simulink library "SimplusGT"  (R2020a)
settings: Solver=ode45  StartTime=0.0  StopTime=10.0  RelTol=1e-3
undefined symbols (not defined in the file): ang_r, Cf, DiscIntNeverNeededParam, initial, Lc, Lf, m, OtherInputs, P_dc, Sbase, t0, Tm_pu, Ts, V, Vbase, w_droop, w_i, w_pll, w_tau, w_v, Wbase, wc, wfil, x0, Ybase, Zbase
libraries: powerlib x307, $bdroot x1, SimplexPS_2015a x1
(part 5 of 7)

== system SimplusGT/SynchronousMachineFull_SMAVRPSS (dq-Frame System Object) ==
  note: Electrical Circuit
  note: Auxiliary
  note: Matlab System Object
  note: Synchronous machine IN Cyprus 14-bus system with AVR, PSS and GOV.
      |
      | Author(s): Yue Zhu
      |
      | Notes:
      |
      | This model is based on matlab system object.
      |
      | The model is in load convention.
      |
      | The frame transformation between dq and abc is done by simulink blocks, i.e., outside the system object.
  note: The actual current with considering discretization
  Bus Creator : BusCreator  Inputs=7
  Constant2 : Constant  Value=OtherInputs
  Constant5 : Constant  Value=2*pi
  Demux : Demux
  Demux1 : Demux  Outputs=3
  Demux2 : Demux  Outputs=2
  Demux3 : Demux  Outputs=2
  Gain : Gain  Gain=1/Wbase
  Gain1 : Gain  Gain=1/Vbase
  Gain2 : Gain  Gain=Sbase/Vbase
  Gain3 : Gain  Gain=1/(Sbase/Vbase)
  MATLAB System1 : MATLABSystem  System=SimplusGT.Class.SynchronousMachineFull_SMAVRPSS  Ts=Ts  Para=ApparatusPara  ApparatusType=ApparatusType  PowerFlow=PowerFlow  x0=x0  DiscreMethod=DiscreMethod  LinearizationTimes=LinearizationTimes  DirectFeedthrough=DirectFeedthrough  VirtualResistor=DiscreDampingFlag  EquiInitial=true  ElecPortIOs=[ 1, 2 ]  SimulateUsing=Code generation
      mask Type: SimplusGT.Class.SynchronousMachineFull_SMAVRPSS
      mask Display:
      | disp('SynchronousMachineFull_SMAVRPSS');
      | port_label('input',1,'u');
      | port_label('output',1,'y');
  Math Function2 : Math  Operator=mod  SignedPower=on  SaturateOnIntegerOverflow=on
  Mux : Mux  Inputs=2
  Mux1 : Mux  Inputs=3
  Mux2 : Mux
  Mux3 : Mux  Inputs=3
  PQ Calculation (dq-Frame) : Subsystem  AncestorBlock=|
      | SimplusGT/PQ Calculation
      | (dq-Frame)
  R_VD : powerlib/Elements/Three-Phase Series RLC Branch  LConnTagsString=A|B|C  RConnTagsString=A|B|C  BranchType=R  Resistance=DiscreDampingValue*Vbase^2/Sbase  Inductance=1e-3  Capacitance=1e-6  Measurements=None
  "abc -> dq (Power-Invariant)" : Subsystem  AncestorBlock=|
      | SimplusGT/abc -> dq
      | (Power-Invariant)
  "abc -> dq (Power-Invariant)1" : Subsystem  AncestorBlock=|
      | SimplusGT/abc -> dq
      | (Power-Invariant)
  "dq -> abc (Power-Invariant)" : Subsystem  AncestorBlock=|
      | SimplusGT/dq -> abc
      | (Power-Invariant)
  ia : powerlib/Electrical Sources/Controlled Current Source  Initialize=on  Source_Type=AC  Amplitude=0  Phase=0  Frequency=0  Measurements=None
  ia_m : powerlib/Measurements/Current Measurement  PhasorSimulation=off  OutputType=Complex  PSBequivalent=0
  ib : powerlib/Electrical Sources/Controlled Current Source  Initialize=on  Source_Type=AC  Amplitude=0  Phase=0  Frequency=0  Measurements=None
  ib_m : powerlib/Measurements/Current Measurement  PhasorSimulation=off  OutputType=Complex  PSBequivalent=0
  ic : powerlib/Electrical Sources/Controlled Current Source  Initialize=on  Source_Type=AC  Amplitude=0  Phase=0  Frequency=0  Measurements=None
  ic_m : powerlib/Measurements/Current Measurement  PhasorSimulation=off  OutputType=Complex  PSBequivalent=0
  va : powerlib/Measurements/Voltage Measurement  PhasorSimulation=off  OutputType=Complex  PSBequivalent=0
  vb : powerlib/Measurements/Voltage Measurement  PhasorSimulation=off  OutputType=Complex  PSBequivalent=0
  vc : powerlib/Measurements/Voltage Measurement  PhasorSimulation=off  OutputType=Complex  PSBequivalent=0
  a : PMIOPort  Side=Left
  b : PMIOPort  Port=2  Side=Left
  c : PMIOPort  Port=3  Side=Left
  n : PMIOPort  Port=4  Side=Left
  m : Outport
  wires:
  "abc -> dq (Power-Invariant)1"/1(dq) -> [i_dq_t]
  [theta] -> "abc -> dq (Power-Invariant)1"/2(theta)
  [i_abc_t] -> "abc -> dq (Power-Invariant)1"/1(abc)
  Gain3/1 -> [i_abc_t]
  Mux3/1 -> Gain3/1
  ic_m/1 -> Mux3/3
  ib_m/1 -> Mux3/2
  ia_m/1 -> Mux3/1
  Gain2/1 -> Demux1/1
  Gain1/1 -> [v_abc]
  [pq] -> Bus Creator/7  "pq"
  PQ Calculation (dq-Frame)/1(pq) -> [pq]
  [i_dq_t] -> PQ Calculation (dq-Frame)/2(idq)  "i_dq"
  [v_dq] -> PQ Calculation (dq-Frame)/1(vdq)  "v_dq"
  [i_abc] -> Gain2/1
  Demux3/2 -> Mux2/4
  Demux3/1 -> Mux2/3
  Constant2/1 -> Demux3/1
  Mux1/1 -> Gain1/1
  Gain/1 -> Bus Creator/5  "w"
  Bus Creator/1 -> m/1
  [theta] -> Bus Creator/6  "theta"
  [w] -> Gain/1  "w"
  [i_abc_t] -> Bus Creator/4  "i_abc"
  [v_abc] -> Bus Creator/3  "v_abc"
  [i_dq_t] -> Bus Creator/2  "i_dq"
  [v_dq] -> Bus Creator/1  "v_dq"
  Math Function2/1 -> [theta]
  Constant5/1 -> Math Function2/2
  Demux/4 -> Math Function2/1
  Demux1/3 -> ic/1
  vc/1 -> Mux1/3
  MATLAB System1/1 -> Demux/1
  Mux2/1 -> MATLAB System1/1
  "dq -> abc (Power-Invariant)"/1(abc) -> [i_abc]
  [theta] -> "dq -> abc (Power-Invariant)"/2(theta)
  [i_dq] -> "dq -> abc (Power-Invariant)"/1(dq)
  "abc -> dq (Power-Invariant)"/1(dq) -> [v_dq]
  [theta] -> "abc -> dq (Power-Invariant)"/2(theta)
  [v_abc] -> "abc -> dq (Power-Invariant)"/1(abc)
  Demux2/2 -> Mux2/2
  Demux2/1 -> Mux2/1
  [v_dq] -> Demux2/1
  vb/1 -> Mux1/2
  va/1 -> Mux1/1
  Demux1/2 -> ib/1
  Demux1/1 -> ia/1
  Demux/3 -> [w]
  Mux/1 -> [i_dq]
  Demux/1 -> Mux/1
  Demux/2 -> Mux/2
  connections:
  ic_m/LConn1 -- c/RConn1
  ib_m/LConn1 -- b/RConn1
  ia_m/LConn1 -- a/RConn1
  ia_m/RConn1 -- ia/LConn1 -- R_VD/LConn1 -- va/LConn1
  vc/LConn1 -- ic_m/RConn1 -- ic/LConn1 -- R_VD/LConn3
  ib/LConn1 -- ib_m/RConn1 -- vb/LConn1 -- R_VD/LConn2
  ic/RConn1 -- n/RConn1 -- ib/RConn1 -- ia/RConn1 -- R_VD/RConn1 -- R_VD/RConn2 -- R_VD/RConn3 -- vc/LConn2 -- va/LConn2 -- vb/LConn2

== system SimplusGT/SynchronousMachineFull_SMAVRPSSGOV (dq-Frame System Object) ==
  note: Electrical Circuit
  note: Auxiliary
  note: Matlab System Object
  note: Synchronous machine IN Cyprus 14-bus system with AVR, PSS and GOV.
      |
      | Author(s): Yue Zhu
      |
      | Notes:
      |
      | This model is based on matlab system object.
      |
      | The model is in load convention.
      |
      | The frame transformation between dq and abc is done by simulink blocks, i.e., outside the system object.
  note: The actual current with considering discretization
  Bus Creator : BusCreator  Inputs=7
  Constant2 : Constant  Value=OtherInputs
  Constant5 : Constant  Value=2*pi
  Demux : Demux
  Demux1 : Demux  Outputs=3
  Demux2 : Demux  Outputs=2
  Demux3 : Demux  Outputs=2
  Gain : Gain  Gain=1/Wbase
  Gain1 : Gain  Gain=1/Vbase
  Gain2 : Gain  Gain=Sbase/Vbase
  Gain3 : Gain  Gain=1/(Sbase/Vbase)
  MATLAB System : MATLABSystem  System=SimplusGT.Class.SynchronousMachineFull_SMAVRPSSGOV  Ts=Ts  Para=ApparatusPara  ApparatusType=ApparatusType  PowerFlow=PowerFlow  x0=x0  DiscreMethod=DiscreMethod  LinearizationTimes=LinearizationTimes  DirectFeedthrough=DirectFeedthrough  VirtualResistor=DiscreDampingFlag  EquiInitial=true  ElecPortIOs=[ 1, 2 ]  SimulateUsing=Code generation
      mask Type: SimplusGT.Class.SynchronousMachineFull_SMAVRPSSGOV
      mask Display:
      | disp('SynchronousMachineFull_SMAVRPSSGOV');
      | port_label('input',1,'u');
      | port_label('output',1,'y');
  Math Function2 : Math  Operator=mod  SignedPower=on  SaturateOnIntegerOverflow=on
  Mux : Mux  Inputs=2
  Mux1 : Mux  Inputs=3
  Mux2 : Mux
  Mux3 : Mux  Inputs=3
  PQ Calculation (dq-Frame) : Subsystem  AncestorBlock=|
      | SimplusGT/PQ Calculation
      | (dq-Frame)
  R_VD : powerlib/Elements/Three-Phase Series RLC Branch  LConnTagsString=A|B|C  RConnTagsString=A|B|C  BranchType=R  Resistance=DiscreDampingValue*Vbase^2/Sbase  Inductance=1e-3  Capacitance=1e-6  Measurements=None
  "abc -> dq (Power-Invariant)" : Subsystem  AncestorBlock=|
      | SimplusGT/abc -> dq
      | (Power-Invariant)
  "abc -> dq (Power-Invariant)1" : Subsystem  AncestorBlock=|
      | SimplusGT/abc -> dq
      | (Power-Invariant)
  "dq -> abc (Power-Invariant)" : Subsystem  AncestorBlock=|
      | SimplusGT/dq -> abc
      | (Power-Invariant)
  ia : powerlib/Electrical Sources/Controlled Current Source  Initialize=on  Source_Type=AC  Amplitude=0  Phase=0  Frequency=0  Measurements=None
  ia_m : powerlib/Measurements/Current Measurement  PhasorSimulation=off  OutputType=Complex  PSBequivalent=0
  ib : powerlib/Electrical Sources/Controlled Current Source  Initialize=on  Source_Type=AC  Amplitude=0  Phase=0  Frequency=0  Measurements=None
  ib_m : powerlib/Measurements/Current Measurement  PhasorSimulation=off  OutputType=Complex  PSBequivalent=0
  ic : powerlib/Electrical Sources/Controlled Current Source  Initialize=on  Source_Type=AC  Amplitude=0  Phase=0  Frequency=0  Measurements=None
  ic_m : powerlib/Measurements/Current Measurement  PhasorSimulation=off  OutputType=Complex  PSBequivalent=0
  va : powerlib/Measurements/Voltage Measurement  PhasorSimulation=off  OutputType=Complex  PSBequivalent=0
  vb : powerlib/Measurements/Voltage Measurement  PhasorSimulation=off  OutputType=Complex  PSBequivalent=0
  vc : powerlib/Measurements/Voltage Measurement  PhasorSimulation=off  OutputType=Complex  PSBequivalent=0
  a : PMIOPort  Side=Left
  b : PMIOPort  Port=2  Side=Left
  c : PMIOPort  Port=3  Side=Left
  n : PMIOPort  Port=4  Side=Left
  m : Outport
  wires:
  "abc -> dq (Power-Invariant)1"/1(dq) -> [i_dq_t]
  [theta] -> "abc -> dq (Power-Invariant)1"/2(theta)
  [i_abc_t] -> "abc -> dq (Power-Invariant)1"/1(abc)
  Gain3/1 -> [i_abc_t]
  Mux3/1 -> Gain3/1
  ic_m/1 -> Mux3/3
  ib_m/1 -> Mux3/2
  ia_m/1 -> Mux3/1
  Gain2/1 -> Demux1/1
  Gain1/1 -> [v_abc]
  [pq] -> Bus Creator/7  "pq"
  PQ Calculation (dq-Frame)/1(pq) -> [pq]
  [i_dq_t] -> PQ Calculation (dq-Frame)/2(idq)  "i_dq"
  [v_dq] -> PQ Calculation (dq-Frame)/1(vdq)  "v_dq"
  [i_abc] -> Gain2/1
  Demux3/2 -> Mux2/4
  Demux3/1 -> Mux2/3
  Constant2/1 -> Demux3/1
  Mux1/1 -> Gain1/1
  Gain/1 -> Bus Creator/5  "w"
  Bus Creator/1 -> m/1
  [theta] -> Bus Creator/6  "theta"
  [w] -> Gain/1  "w"
  [i_abc_t] -> Bus Creator/4  "i_abc"
  [v_abc] -> Bus Creator/3  "v_abc"
  [i_dq_t] -> Bus Creator/2  "i_dq"
  [v_dq] -> Bus Creator/1  "v_dq"
  Math Function2/1 -> [theta]
  Constant5/1 -> Math Function2/2
  Demux/4 -> Math Function2/1
  Demux1/3 -> ic/1
  vc/1 -> Mux1/3
  MATLAB System/1 -> Demux/1
  Mux2/1 -> MATLAB System/1
  "dq -> abc (Power-Invariant)"/1(abc) -> [i_abc]
  [theta] -> "dq -> abc (Power-Invariant)"/2(theta)
  [i_dq] -> "dq -> abc (Power-Invariant)"/1(dq)
  "abc -> dq (Power-Invariant)"/1(dq) -> [v_dq]
  [theta] -> "abc -> dq (Power-Invariant)"/2(theta)
  [v_abc] -> "abc -> dq (Power-Invariant)"/1(abc)
  Demux2/2 -> Mux2/2
  Demux2/1 -> Mux2/1
  [v_dq] -> Demux2/1
  vb/1 -> Mux1/2
  va/1 -> Mux1/1
  Demux1/2 -> ib/1
  Demux1/1 -> ia/1
  Demux/3 -> [w]
  Mux/1 -> [i_dq]
  Demux/1 -> Mux/1
  Demux/2 -> Mux/2
  connections:
  ic_m/LConn1 -- c/RConn1
  ib_m/LConn1 -- b/RConn1
  ia_m/LConn1 -- a/RConn1
  ia_m/RConn1 -- ia/LConn1 -- R_VD/LConn1 -- va/LConn1
  vc/LConn1 -- ic_m/RConn1 -- ic/LConn1 -- R_VD/LConn3
  ib/LConn1 -- ib_m/RConn1 -- vb/LConn1 -- R_VD/LConn2
  ic/RConn1 -- n/RConn1 -- ib/RConn1 -- ia/RConn1 -- R_VD/RConn1 -- R_VD/RConn2 -- R_VD/RConn3 -- vc/LConn2 -- va/LConn2 -- vb/LConn2

== system SimplusGT/SynchronousMachineFull_SM_GOV (dq-Frame System Object) ==
  note: Electrical Circuit
  note: Auxiliary
  note: Matlab System Object
  note: Synchronous machine IN Cyprus 14-bus system with AVR, PSS and GOV.
      |
      | Author(s): Yue Zhu
      |
      | Notes:
      |
      | This model is based on matlab system object.
      |
      | The model is in load convention.
      |
      | The frame transformation between dq and abc is done by simulink blocks, i.e., outside the system object.
  note: The actual current with considering discretization
  Bus Creator : BusCreator  Inputs=7
  Constant2 : Constant  Value=OtherInputs
  Constant5 : Constant  Value=2*pi
  Demux : Demux
  Demux1 : Demux  Outputs=3
  Demux2 : Demux  Outputs=2
  Demux3 : Demux  Outputs=2
  Gain : Gain  Gain=1/Wbase
  Gain1 : Gain  Gain=1/Vbase
  Gain2 : Gain  Gain=Sbase/Vbase
  Gain3 : Gain  Gain=1/(Sbase/Vbase)
  MATLAB System : MATLABSystem  System=SimplusGT.Class.SynchronousMachineFull_SM_GOV  Ts=Ts  Para=ApparatusPara  ApparatusType=ApparatusType  PowerFlow=PowerFlow  x0=x0  DiscreMethod=DiscreMethod  LinearizationTimes=LinearizationTimes  DirectFeedthrough=DirectFeedthrough  VirtualResistor=DiscreDampingFlag  EquiInitial=true  ElecPortIOs=[ 1, 2 ]  SimulateUsing=Code generation
      mask Type: SimplusGT.Class.SynchronousMachineFull_SM_GOV
      mask Display:
      | disp('SynchronousMachineFull_SM_GOV');
      | port_label('input',1,'u');
      | port_label('output',1,'y');
  Math Function2 : Math  Operator=mod  SignedPower=on  SaturateOnIntegerOverflow=on
  Mux : Mux  Inputs=2
  Mux1 : Mux  Inputs=3
  Mux2 : Mux
  Mux3 : Mux  Inputs=3
  PQ Calculation (dq-Frame) : Subsystem  AncestorBlock=|
      | SimplusGT/PQ Calculation
      | (dq-Frame)
  R_VD : powerlib/Elements/Three-Phase Series RLC Branch  LConnTagsString=A|B|C  RConnTagsString=A|B|C  BranchType=R  Resistance=DiscreDampingValue*Vbase^2/Sbase  Inductance=1e-3  Capacitance=1e-6  Measurements=None
  "abc -> dq (Power-Invariant)" : Subsystem  AncestorBlock=|
      | SimplusGT/abc -> dq
      | (Power-Invariant)
  "abc -> dq (Power-Invariant)1" : Subsystem  AncestorBlock=|
      | SimplusGT/abc -> dq
      | (Power-Invariant)
  "dq -> abc (Power-Invariant)" : Subsystem  AncestorBlock=|
      | SimplusGT/dq -> abc
      | (Power-Invariant)
  ia : powerlib/Electrical Sources/Controlled Current Source  Initialize=on  Source_Type=AC  Amplitude=0  Phase=0  Frequency=0  Measurements=None
  ia_m : powerlib/Measurements/Current Measurement  PhasorSimulation=off  OutputType=Complex  PSBequivalent=0
  ib : powerlib/Electrical Sources/Controlled Current Source  Initialize=on  Source_Type=AC  Amplitude=0  Phase=0  Frequency=0  Measurements=None
  ib_m : powerlib/Measurements/Current Measurement  PhasorSimulation=off  OutputType=Complex  PSBequivalent=0
  ic : powerlib/Electrical Sources/Controlled Current Source  Initialize=on  Source_Type=AC  Amplitude=0  Phase=0  Frequency=0  Measurements=None
  ic_m : powerlib/Measurements/Current Measurement  PhasorSimulation=off  OutputType=Complex  PSBequivalent=0
  va : powerlib/Measurements/Voltage Measurement  PhasorSimulation=off  OutputType=Complex  PSBequivalent=0
  vb : powerlib/Measurements/Voltage Measurement  PhasorSimulation=off  OutputType=Complex  PSBequivalent=0
  vc : powerlib/Measurements/Voltage Measurement  PhasorSimulation=off  OutputType=Complex  PSBequivalent=0
  a : PMIOPort  Side=Left
  b : PMIOPort  Port=2  Side=Left
  c : PMIOPort  Port=3  Side=Left
  n : PMIOPort  Port=4  Side=Left
  m : Outport
  wires:
  "abc -> dq (Power-Invariant)1"/1(dq) -> [i_dq_t]
  [theta] -> "abc -> dq (Power-Invariant)1"/2(theta)
  [i_abc_t] -> "abc -> dq (Power-Invariant)1"/1(abc)
  Gain3/1 -> [i_abc_t]
  Mux3/1 -> Gain3/1
  ic_m/1 -> Mux3/3
  ib_m/1 -> Mux3/2
  ia_m/1 -> Mux3/1
  Gain2/1 -> Demux1/1
  Gain1/1 -> [v_abc]
  [pq] -> Bus Creator/7  "pq"
  PQ Calculation (dq-Frame)/1(pq) -> [pq]
  [i_dq_t] -> PQ Calculation (dq-Frame)/2(idq)  "i_dq"
  [v_dq] -> PQ Calculation (dq-Frame)/1(vdq)  "v_dq"
  [i_abc] -> Gain2/1
  Demux3/2 -> Mux2/4
  Demux3/1 -> Mux2/3
  Constant2/1 -> Demux3/1
  Mux1/1 -> Gain1/1
  Gain/1 -> Bus Creator/5  "w"
  Bus Creator/1 -> m/1
  [theta] -> Bus Creator/6  "theta"
  [w] -> Gain/1  "w"
  [i_abc_t] -> Bus Creator/4  "i_abc"
  [v_abc] -> Bus Creator/3  "v_abc"
  [i_dq_t] -> Bus Creator/2  "i_dq"
  [v_dq] -> Bus Creator/1  "v_dq"
  Math Function2/1 -> [theta]
  Constant5/1 -> Math Function2/2
  Demux/4 -> Math Function2/1
  Demux1/3 -> ic/1
  vc/1 -> Mux1/3
  MATLAB System/1 -> Demux/1
  Mux2/1 -> MATLAB System/1
  "dq -> abc (Power-Invariant)"/1(abc) -> [i_abc]
  [theta] -> "dq -> abc (Power-Invariant)"/2(theta)
  [i_dq] -> "dq -> abc (Power-Invariant)"/1(dq)
  "abc -> dq (Power-Invariant)"/1(dq) -> [v_dq]
  [theta] -> "abc -> dq (Power-Invariant)"/2(theta)
  [v_abc] -> "abc -> dq (Power-Invariant)"/1(abc)
  Demux2/2 -> Mux2/2
  Demux2/1 -> Mux2/1
  [v_dq] -> Demux2/1
  vb/1 -> Mux1/2
  va/1 -> Mux1/1
  Demux1/2 -> ib/1
  Demux1/1 -> ia/1
  Demux/3 -> [w]
  Mux/1 -> [i_dq]
  Demux/1 -> Mux/1
  Demux/2 -> Mux/2
  connections:
  ic_m/LConn1 -- c/RConn1
  ib_m/LConn1 -- b/RConn1
  ia_m/LConn1 -- a/RConn1
  ia_m/RConn1 -- ia/LConn1 -- R_VD/LConn1 -- va/LConn1
  vc/LConn1 -- ic_m/RConn1 -- ic/LConn1 -- R_VD/LConn3
  ib/LConn1 -- ib_m/RConn1 -- vb/LConn1 -- R_VD/LConn2
  ic/RConn1 -- n/RConn1 -- ib/RConn1 -- ia/RConn1 -- R_VD/RConn1 -- R_VD/RConn2 -- R_VD/RConn3 -- vc/LConn2 -- va/LConn2 -- vb/LConn2

== system SimplusGT/Three-Phase Bus ==
  note: Electrical Circuit
  note: Model for a three-phase bus.
      |
      | Author(s): Yitong Li
      |
      | Notes:
      |
      | It is simply a short-cuirt with current measurement. It is used in the toolbox model for highlighting the position of a bus and making the layout clearer.
  Mux : Mux  Inputs=3
  ia : powerlib/Measurements/Current Measurement  PhasorSimulation=off  OutputType=Complex  PSBequivalent=0
  ib : powerlib/Measurements/Current Measurement  PhasorSimulation=off  OutputType=Complex  PSBequivalent=0
  ic : powerlib/Measurements/Current Measurement  PhasorSimulation=off  OutputType=Complex  PSBequivalent=0
  a+ : PMIOPort  Side=Left
  -a : PMIOPort  Port=2  Side=Right
  b+ : PMIOPort  Port=3  Side=Left
  -b : PMIOPort  Port=4  Side=Right
  c+ : PMIOPort  Port=5  Side=Left
  -c : PMIOPort  Port=6  Side=Right
  wires:
  Mux/1 -> [iabc]
  ia/1 -> Mux/1
  ib/1 -> Mux/2
  ic/1 -> Mux/3
  connections:
  ic/RConn1 -- -c/RConn1
  ib/LConn1 -- b+/RConn1
  ib/RConn1 -- -b/RConn1
  ic/LConn1 -- c+/RConn1
  ia/LConn1 -- a+/RConn1
  ia/RConn1 -- -a/RConn1

== system SimplusGT/Three-Phase Signal ==
  note: Three-phase signal generator
      |
      | Author(s): Yitong Li
  Constant : Constant  Value=[ud uq]
  Constant1 : Constant  Value=w
  Constant2 : Constant  Value=theta0
  Constant3 : Constant  Value=2*pi
  Discrete-Time Integrator : DiscreteIntegrator  InitialConditionSource=external  SampleTime=Ts  ICPrevOutput=DiscIntNeverNeededParam  ICPrevScaledInput=DiscIntNeverNeededParam
  Math Function1 : Math  Operator=mod  SignedPower=on  SaturateOnIntegerOverflow=on
  "dq -> abc (Power-Invariant)" : Subsystem
  abc : Outport
  dq : Outport  Port=2
  theta : Outport  Port=3
  wires:
  Discrete-Time Integrator/1 -> Math Function1/1
  "dq -> abc (Power-Invariant)"/1(abc) -> abc/1
  Constant/1 -> "dq -> abc (Power-Invariant)"/1(dq), dq/1
  Math Function1/1 -> "dq -> abc (Power-Invariant)"/2(theta), theta/1
  Constant3/1 -> Math Function1/2
  Constant2/1 -> Discrete-Time Integrator/2
  Constant1/1 -> Discrete-Time Integrator/1

== system SimplusGT/Three-Phase Signal (Advanced) ==
  note: Three-phase signal generator
      |
      | Author(s): Yitong Li
      |
      | Notes:
      |
      | This block has advanced settings.
  Constant : Constant  Value=[ud uq]
  Constant1 : Constant  Value=w
  Constant2 : Constant  Value=theta0
  Constant3 : Constant  Value=2*pi
  Constant4 : Constant  Value=enable_freq_step
  Discrete-Time Integrator : DiscreteIntegrator  InitialConditionSource=external  SampleTime=Ts  ICPrevOutput=DiscIntNeverNeededParam  ICPrevScaledInput=DiscIntNeverNeededParam
  Math Function1 : Math  Operator=mod  SignedPower=on  SaturateOnIntegerOverflow=on
  Product : Product
  Step : Step  Time=time_freq_step  Before=1  After=ratio_freq_step  SampleTime=0
  Switch : Switch  Criteria=u2 > Threshold  Threshold=0.5
  "dq -> abc (Power-Invariant)1" : SimplexPS_2015a/Three-Phase Signal/dq -> abc (Power-Invariant)  SystemSampleTime=-1  Latency=0  AutoFrameSizeCalculation=off
  abc : Outport
  dq : Outport  Port=2
  theta : Outport  Port=3
  wires:
  Constant3/1 -> Math Function1/2
  Constant4/1 -> Switch/2
  Switch/1 -> Discrete-Time Integrator/1
  Constant1/1 -> Product/2, Switch/3
  Constant2/1 -> Discrete-Time Integrator/2
  Product/1 -> Switch/1
  Math Function1/1 -> theta/1, "dq -> abc (Power-Invariant)1"/2
  Constant/1 -> dq/1, "dq -> abc (Power-Invariant)1"/1
  Discrete-Time Integrator/1 -> Math Function1/1
  "dq -> abc (Power-Invariant)1"/1 -> abc/1
  Step/1 -> Product/1

== system SimplusGT/Timer ==
  note: Timer
      |
      | Author(s): Yitong Li
  Constant : Constant
  Discrete-Time Integrator : DiscreteIntegrator  SampleTime=Ts  ICPrevOutput=DiscIntNeverNeededParam  ICPrevScaledInput=DiscIntNeverNeededParam
  Gain : Gain
  Gain1 : Gain  Gain=1/60
  Gain2 : Gain  Gain=1/60
  sec : Outport
  min : Outport  Port=2
  h : Outport  Port=3
  wires:
  Constant/1 -> Discrete-Time Integrator/1
  Discrete-Time Integrator/1 -> Gain/1
  Gain/1 -> Gain1/1, sec/1
  Gain1/1 -> Gain2/1, min/1
  Gain2/1 -> h/1

== system SimplusGT/Two-Phase Bus ==
  note: Electrical Circuit
  note: Model for a two-phase bus.
      |
      | Author(s): Yitong Li
      |
      | Notes:
      |
      | It is simply a short-cuirt with current measurement. It is used in the toolbox model for highlighting the position of a bus and making the layout clearer.
  Mux : Mux  Inputs=2
  ia : powerlib/Measurements/Current Measurement  PhasorSimulation=off  OutputType=Complex  PSBequivalent=0
  ib : powerlib/Measurements/Current Measurement  PhasorSimulation=off  OutputType=Complex  PSBequivalent=0
  a+ : PMIOPort  Side=Left
  -a : PMIOPort  Port=2  Side=Right
  b+ : PMIOPort  Port=3  Side=Left
  -b : PMIOPort  Port=4  Side=Right
  wires:
  Mux/1 -> [iab]
  ia/1 -> Mux/1
  ib/1 -> Mux/2
  connections:
  ib/LConn1 -- b+/RConn1
  ib/RConn1 -- -b/RConn1
  ia/LConn1 -- a+/RConn1
  ia/RConn1 -- -a/RConn1

== system SimplusGT/Voltage Measurement (2ph -> 3ph) ==
  note: Three-phase voltage measurement.
      |
      | Author(s): Yitong Li
      |
      | Notes:
      |
      | vc is calculated from va and vb with assuming that va + vb + vc = 0.
  Add : Sum  Inputs=--+
  Constant : Constant  Value=0
  Mux : Mux  Inputs=3
  va : powerlib/Measurements/Voltage Measurement  PhasorSimulation=off  OutputType=Complex  PSBequivalent=0
  vb : powerlib/Measurements/Voltage Measurement  PhasorSimulation=off  OutputType=Complex  PSBequivalent=0
  a : PMIOPort  Side=Left
  b : PMIOPort  Port=2  Side=Left
  n : PMIOPort  Port=3  Side=Left
  vabc : Outport
  wires:
  Mux/1 -> vabc/1
  va/1 -> Mux/1, Add/1
  vb/1 -> Mux/2, Add/2
  Constant/1 -> Add/3
  Add/1 -> Mux/3
  connections:
  vb/LConn2 -- va/LConn2 -- n/RConn1
  vb/LConn1 -- b/RConn1
  va/LConn1 -- a/RConn1

== system SimplusGT/Voltage Measurement (3ph -> 3ph) ==
  note: Three-phase voltage measurement.
      |
      | Author(s): Yitong Li
  Mux : Mux  Inputs=3
  va : powerlib/Measurements/Voltage Measurement  PhasorSimulation=off  OutputType=Complex  PSBequivalent=0
  vb : powerlib/Measurements/Voltage Measurement  PhasorSimulation=off  OutputType=Complex  PSBequivalent=0
  vc : powerlib/Measurements/Voltage Measurement  PhasorSimulation=off  OutputType=Complex  PSBequivalent=0
  a : PMIOPort  Side=Left
  b : PMIOPort  Port=2  Side=Left
  c : PMIOPort  Port=3  Side=Left
  n : PMIOPort  Port=4  Side=Left
  vabc : Outport
  wires:
  vc/1 -> Mux/3
  Mux/1 -> vabc/1
  va/1 -> Mux/1
  vb/1 -> Mux/2
  connections:
  vb/LConn2 -- va/LConn2 -- vc/LConn2 -- n/RConn1
  vc/LConn1 -- c/RConn1
  vb/LConn1 -- b/RConn1
  va/LConn1 -- a/RConn1

== system SimplusGT/Voltage Disturbance ==
  note: Model for a voltage disturbance.
      |
      | Author(s): Yitong Li
  vabc : Inport
  Controlled Voltage Source : powerlib/Electrical Sources/Controlled Voltage Source  Initialize=on  Source_Type=AC  Amplitude=0  Phase=0  Frequency=0  Measurements=None
  Controlled Voltage Source1 : powerlib/Electrical Sources/Controlled Voltage Source  Initialize=on  Source_Type=AC  Amplitude=0  Phase=0  Frequency=0  Measurements=None
  Controlled Voltage Source2 : powerlib/Electrical Sources/Controlled Voltage Source  Initialize=on  Source_Type=AC  Amplitude=0  Phase=0  Frequency=0  Measurements=None
  Demux : Demux  Outputs=3
  Gain : Gain  Gain=Vbase
  a+ : PMIOPort  Side=Right
  a- : PMIOPort  Port=2  Side=Left
  b+ : PMIOPort  Port=3  Side=Right
  b- : PMIOPort  Port=4  Side=Left
  c+ : PMIOPort  Port=5  Side=Right
  c- : PMIOPort  Port=6  Side=Left
  wires:
  vabc/1 -> Gain/1
  Demux/1 -> Controlled Voltage Source/1
  Demux/2 -> Controlled Voltage Source1/1
  Demux/3 -> Controlled Voltage Source2/1
  Gain/1 -> Demux/1
  connections:
  Controlled Voltage Source2/LConn1 -- c-/RConn1
  Controlled Voltage Source1/RConn1 -- b+/RConn1
  Controlled Voltage Source2/RConn1 -- c+/RConn1
  Controlled Voltage Source/RConn1 -- a+/RConn1
  Controlled Voltage Source/LConn1 -- a-/RConn1
  Controlled Voltage Source1/LConn1 -- b-/RConn1

== system SimplusGT/abc -> alpha//beta (Power-Invariant) ==
  note: Frame transformation from abc to alpha/beta.
      |
      | Author(s): Yitong Li
      |
      | Notes:
      |
      | The transformation is power-invariant.
  abc : Inport
  ->alpha : Fcn  Expr=u(1) - 1/2*u(2) - 1/2*u(3)
  ->beta : Fcn  Expr=0 + sqrt(3)/2*u(2) - sqrt(3)/2*u(3)
  Gain : Gain  Gain=sqrt(2/3)
  Mux2 : Mux  Inputs=2
  albe : Outport
  wires:
  abc/1 -> Gain/1
  Mux2/1 -> albe/1
  Gain/1 -> ->alpha/1, ->beta/1
  ->alpha/1 -> Mux2/1
  ->beta/1 -> Mux2/2

== system SimplusGT/abc -> alpha//beta//0 (Power-Invariant) ==
  note: Frame transformation from abc to alpha/beta/0.
      |
      | Author(s): Yitong Li
      |
      | Notes:
      |
      | The transformation is power-invariant.
  abc : Inport
  ->0 : Fcn  Expr=1/sqrt(2)*u(1) + 1/sqrt(2)*u(2) + 1/sqrt(2)*u(3)
  ->alpha : Fcn  Expr=u(1) - 1/2*u(2) - 1/2*u(3)
  ->beta : Fcn  Expr=0 + sqrt(3)/2*u(2) - sqrt(3)/2*u(3)
  Gain : Gain  Gain=sqrt(2/3)
  Mux2 : Mux  Inputs=3
  albe0 : Outport
  wires:
  ->beta/1 -> Mux2/2
  ->alpha/1 -> Mux2/1
  Gain/1 -> ->alpha/1, ->0/1, ->beta/1
  Mux2/1 -> albe0/1
  abc/1 -> Gain/1
  ->0/1 -> Mux2/3

== system SimplusGT/abc -> dq (Power-Invariant) ==
  note: Frame transformation from abc to dq.
      |
      | Author(s): Yitong Li
      |
      | Notes:
      |
      | The transformation is power-invariant.
      |
      | theta is the angle that d axis leads a axis.
      |
      | q axis leads d axis by 90 degrees.
  abc : Inport
  theta : Inport  Port=2
  ->d : Fcn  Expr=cos(u(4))*u(1) + cos(u(4)-2/3*pi)*u(2) + cos(u(4)-4/3*pi)*u(3)
  ->q : Fcn  Expr=-sin(u(4))*u(1) - sin(u(4)-2/3*pi)*u(2) - sin(u(4)-4/3*pi)*u(3)
  Gain : Gain  Gain=sqrt(2/3)
  Mux5 : Mux  Inputs=2
  Mux6 : Mux  Inputs=2
  dq : Outport
  wires:
  Mux5/1 -> ->q/1, ->d/1
  Mux6/1 -> dq/1
  ->q/1 -> Mux6/2
  theta/1 -> Mux5/2
  Gain/1 -> Mux5/1
  ->d/1 -> Mux6/1
  abc/1 -> Gain/1

== system SimplusGT/abc -> dq (Power-Invariant) (Complex Theta) ==
  abc : Inport
  theta+ : Inport  Port=2
  ->d : Fcn  Expr=cos(u(4))*u(1) + cos(u(4)-2/3*pi)*u(2) + cos(u(4)-4/3*pi)*u(3)
  ->q : Fcn  Expr=-sin(u(4))*u(1) - sin(u(4)-2/3*pi)*u(2) - sin(u(4)-4/3*pi)*u(3)
  Complex to Real-Imag : ComplexToRealImag
  Gain : Gain  Gain=sqrt(2/3)
  Math Function : Math  SignedPower=on  SaturateOnIntegerOverflow=on
  Mux5 : Mux  Inputs=2
  Mux6 : Mux  Inputs=2
  Product : Product
  dq : Outport
  wires:
  ->q/1 -> Mux6/2
  abc/1 -> Gain/1
  Mux5/1 -> ->q/1, ->d/1
  Mux6/1 -> dq/1
  ->d/1 -> Mux6/1
  theta+/1 -> Complex to Real-Imag/1
  Complex to Real-Imag/1 -> Mux5/2
  Complex to Real-Imag/2 -> Math Function/1
  Gain/1 -> Product/1
  Product/1 -> Mux5/1
  Math Function/1 -> Product/2

== system SimplusGT/abc -> dq0 (Power-Invariant) ==
  note: Frame transformation from abc to dq0.
      |
      | Author(s): Yitong Li
      |
      | Notes:
      |
      | The transformation is power-invariant.
      |
      | theta is the angle that dq axis leads abc axis, specifically, d axis leads a axis.
      |
      | q axis leads d axis by 90 degrees. b leads a axis 90 degrees. c leads b 90 degrees.
  abc : Inport
  theta : Inport  Port=2
  ->0 : Fcn  Expr=sqrt(2)/2*u(1) + sqrt(2)/2*u(2) + sqrt(2)/2*u(3)
  ->d : Fcn  Expr=cos(u(4))*u(1) + cos(u(4)-2/3*pi)*u(2) + cos(u(4)-4/3*pi)*u(3)
  ->q : Fcn  Expr=-sin(u(4))*u(1) - sin(u(4)-2/3*pi)*u(2) - sin(u(4)-4/3*pi)*u(3)
  Gain : Gain  Gain=sqrt(2/3)
  Mux1 : Mux  Inputs=2
  Mux2 : Mux  Inputs=3
  dq0 : Outport
  wires:
  ->d/1 -> Mux2/1
  ->q/1 -> Mux2/2
  Gain/1 -> Mux1/1
  abc/1 -> Gain/1
  theta/1 -> Mux1/2
  Mux1/1 -> ->0/1, ->d/1, ->q/1
  Mux2/1 -> dq0/1
  ->0/1 -> Mux2/3

== system SimplusGT/abc->dq (Power-Invariant) (theta_dq) ==
  abc : Inport
  theta_dq : Inport  Port=2
  ->d : Fcn  Expr=cos(u(4))*u(1) + cos(u(4)-2/3*pi)*u(2) + cos(u(4)-4/3*pi)*u(3)
  ->q : Fcn  Expr=-sin(u(4))*u(1) - sin(u(4)-2/3*pi)*u(2) - sin(u(4)-4/3*pi)*u(3)
  Demux : Demux  Outputs=2
  Gain : Gain  Gain=sqrt(2/3)
  Math Function : Math  SignedPower=on  SaturateOnIntegerOverflow=on
  Mux5 : Mux  Inputs=2
  Mux6 : Mux  Inputs=2
  Product : Product
  dq : Outport
  wires:
  Gain/1 -> Product/1
  Math Function/1 -> Product/2
  Mux6/1 -> dq/1
  Mux5/1 -> ->q/1, ->d/1
  ->d/1 -> Mux6/1
  Product/1 -> Mux5/1
  abc/1 -> Gain/1
  ->q/1 -> Mux6/2
  theta_dq/1 -> Demux/1
  Demux/1 -> Mux5/2
  Demux/2 -> Math Function/1

== system SimplusGT/alpha//beta -> abc (Power-Invariant) ==
  note: Frame transformation from alpha/beta to abc.
      |
      | Author(s): Yitong Li
      |
      | Notes:
      |
      | The transformation is power-invariant.
  albe : Inport
  ->a : Fcn  Expr=u(1) + 0
  ->b : Fcn  Expr=-1/2*u(1) + sqrt(3)/2*u(2)
  ->c : Fcn  Expr=-1/2*u(1) - sqrt(3)/2*u(2)
  Gain : Gain  Gain=sqrt(2/3)
  Mux2 : Mux  Inputs=3
  abc : Outport
  wires:
  Gain/1 -> ->a/1, ->c/1, ->b/1
  Mux2/1 -> abc/1
  ->c/1 -> Mux2/3
  ->b/1 -> Mux2/2
  ->a/1 -> Mux2/1
  albe/1 -> Gain/1

== system SimplusGT/alpha//beta -> dq ==
  note: Frame transformation from alpha/beta to dq.
      |
      | Author(s): Yitong Li
      |
      | Notes:
      |
      | theta is the angle that dq axis leads alpha/beta axis, specifically, d axis leads alpha axis.
  albe : Inport
  theta : Inport  Port=2
  ->d : Fcn  Expr=cos(u(3))*u(1) + sin(u(3))*u(2)
  ->q : Fcn  Expr=-sin(u(3))*u(1) + cos(u(3))*u(2)
  Mux5 : Mux  Inputs=2
  Mux6 : Mux  Inputs=2
  dq : Outport
  wires:
  Mux5/1 -> ->q/1, ->d/1
  albe/1 -> Mux5/1
  theta/1 -> Mux5/2
  Mux6/1 -> dq/1
  ->q/1 -> Mux6/2
  ->d/1 -> Mux6/1

== system SimplusGT/alpha//beta//0 -> abc (Power-Invariant) ==
  note: Frame transformation from alpha/beta0 to abc.
      |
      | Author(s): Yitong Li
      |
      | Notes:
      |
      | The transformation is power-invariant.
  albe0 : Inport
  ->a : Fcn  Expr=u(1) + 0 + 1/sqrt(2)*u(3)
  ->b : Fcn  Expr=-1/2*u(1) + sqrt(3)/2*u(2) + 1/sqrt(2)*u(3)
  ->c : Fcn  Expr=-1/2*u(1) - sqrt(3)/2*u(2) + 1/sqrt(2)*u(3)
  Gain : Gain  Gain=sqrt(2/3)
  Mux2 : Mux  Inputs=3
  abc : Outport
  wires:
  Gain/1 -> ->a/1, ->c/1, ->b/1
  ->c/1 -> Mux2/3
  albe0/1 -> Gain/1
  ->a/1 -> Mux2/1
  ->b/1 -> Mux2/2
  Mux2/1 -> abc/1

== system SimplusGT/dq -> abc (Power-Invariant) ==
  note: Frame transformation from dq to abc.
      |
      | Author(s): Yitong Li
      |
      | Notes:
      |
      | The transformation is power-invariant.
      |
      | theta is the angle that dq axis leads alpha/beta axis, specifically, d axis leads alpha axis.
  dq : Inport
  theta : Inport  Port=2
  ->a : Fcn  Expr=cos(u(3))*u(1) - sin(u(3))*u(2)
  ->b : Fcn  Expr=cos(u(3)-2/3*pi)*u(1) - sin(u(3)-2/3*pi)*u(2)
  ->c : Fcn  Expr=cos(u(3)-4/3*pi)*u(1) - sin(u(3)-4/3*pi)*u(2)
  Gain : Gain  Gain=sqrt(2/3)
  Mux5 : Mux  Inputs=2
  Mux6 : Mux  Inputs=3
  abc : Outport
  wires:
  theta/1 -> Mux5/2
  Mux5/1 -> ->c/1, ->a/1, ->b/1
  Mux6/1 -> abc/1
  ->c/1 -> Mux6/3
  dq/1 -> Gain/1
  Gain/1 -> Mux5/1
  ->a/1 -> Mux6/1
  ->b/1 -> Mux6/2

== system SimplusGT/dq -> abc (Power-Invariant) (Complex Theta) ==
  dq : Inport
  theta+ : Inport  Port=2
  ->a : Fcn  Expr=cos(u(3))*u(1) - sin(u(3))*u(2)
  ->b : Fcn  Expr=cos(u(3)-2/3*pi)*u(1) - sin(u(3)-2/3*pi)*u(2)
  ->c : Fcn  Expr=cos(u(3)-4/3*pi)*u(1) - sin(u(3)-4/3*pi)*u(2)
  Complex to Real-Imag : ComplexToRealImag
  Gain : Gain  Gain=sqrt(2/3)
  Gain1 : Gain  Gain=-1
  Math Function : Math  SignedPower=on  SaturateOnIntegerOverflow=on
  Mux5 : Mux  Inputs=2
  Mux6 : Mux  Inputs=3
  Product : Product
  abc : Outport
  wires:
  ->b/1 -> Mux6/2
  ->a/1 -> Mux6/1
  dq/1 -> Gain/1
  ->c/1 -> Mux6/3
  Mux6/1 -> abc/1
  Mux5/1 -> ->c/1, ->a/1, ->b/1
  theta+/1 -> Complex to Real-Imag/1
  Math Function/1 -> Product/2
  Complex to Real-Imag/1 -> Mux5/2
  Product/1 -> Mux5/1
  Gain/1 -> Product/1
  Complex to Real-Imag/2 -> Gain1/1
  Gain1/1 -> Math Function/1

== system SimplusGT/dq->abc (Power-Invariant) (theta_dq) ==
  dq : Inport
  theta_dq : Inport  Port=2
  ->a : Fcn  Expr=cos(u(3))*u(1) - sin(u(3))*u(2)
  ->b : Fcn  Expr=cos(u(3)-2/3*pi)*u(1) - sin(u(3)-2/3*pi)*u(2)
  ->c : Fcn  Expr=cos(u(3)-4/3*pi)*u(1) - sin(u(3)-4/3*pi)*u(2)
  Demux : Demux  Outputs=2
  Gain : Gain  Gain=sqrt(2/3)
  Gain1 : Gain  Gain=-1
  Math Function : Math  SignedPower=on  SaturateOnIntegerOverflow=on
  Mux5 : Mux  Inputs=2
  Mux6 : Mux  Inputs=3
  Product : Product
  abc : Outport
  wires:
  Mux6/1 -> abc/1
  Demux/1 -> Mux5/2
  Product/1 -> Mux5/1
  ->a/1 -> Mux6/1
  Gain1/1 -> Math Function/1
  Math Function/1 -> Product/2
  ->c/1 -> Mux6/3
  Mux5/1 -> ->c/1, ->a/1, ->b/1
  ->b/1 -> Mux6/2
  theta_dq/1 -> Demux/1
  Gain/1 -> Product/1
  dq/1 -> Gain/1
  Demux/2 -> Gain1/1

== system SimplusGT/dq0 -> abc (Power-Invariant) ==
  note: Frame transformation from dq0 to abc.
      |
      | Author(s): Yitong Li
      |
      | Notes:
      |
      | The transformation is power-invariant.
      |
      | theta is the angle that dq axis leads alpha/beta axis, specifically, d axis leads alpha axis.
  dq0 : Inport
  theta : Inport  Port=2
  ->a : Fcn  Expr=cos(u(4))*u(1) - sin(u(4))*u(2) + sqrt(2)/2*u(3)
  ->b : Fcn  Expr=cos(u(4)-2/3*pi)*u(1) - sin(u(4)-2/3*pi)*u(2) + sqrt(2)/2*u(3)
  ->c : Fcn  Expr=cos(u(4)-4/3*pi)*u(1) - sin(u(4)-4/3*pi)*u(2) + sqrt(2)/2*u(3)
  Gain : Gain  Gain=sqrt(2/3)
  Mux1 : Mux  Inputs=2
  Mux2 : Mux  Inputs=3
  abc : Outport
  wires:
  ->a/1 -> Mux2/1
  ->b/1 -> Mux2/2
  Gain/1 -> Mux1/1
  dq0/1 -> Gain/1
  theta/1 -> Mux1/2
  Mux1/1 -> ->c/1, ->a/1, ->b/1
  Mux2/1 -> abc/1
  ->c/1 -> Mux2/3

== system SimplusGT/x1y1 -> x2y2 ==
  note: Frame transformation from x1y1 to x2y2.
      |
      | Author(s): Yitong Li
      |
      | Notes:
      |
      | theta is the phase angle that coordinate 2 (axis) leads coordinate 1 (axis).
  x1y1 : Inport
  theta : Inport  Port=2
  ->x2 : Fcn  Expr=cos(u(3))*u(1) + sin(u(3))*u(2)
  ->y2 : Fcn  Expr=-sin(u(3))*u(1) + cos(u(3))*u(2)
  Mux5 : Mux  Inputs=2
  Mux6 : Mux  Inputs=2
  x2y2 : Outport
  wires:
  Mux6/1 -> x2y2/1
  Mux5/1 -> ->y2/1, ->x2/1
  theta/1 -> Mux5/2
  x1y1/1 -> Mux5/1
  ->y2/1 -> Mux6/2
  ->x2/1 -> Mux6/1

== system SimplusGT/x2y2 -> x1y1 ==
  note: Frame transformation from x2y2 to x1y1.
      |
      | Author(s): Yitong Li
      |
      | Notes:
      |
      | theta is the phase angle that coordinate 2 (axis) leads coordinate 1 (axis).
  x2y2 : Inport
  theta : Inport  Port=2
  ->x2 : Fcn  Expr=cos(u(3))*u(1) - sin(u(3))*u(2)
  ->y2 : Fcn  Expr=sin(u(3))*u(1) + cos(u(3))*u(2)
  Mux5 : Mux  Inputs=2
  Mux6 : Mux  Inputs=2
  x1y1 : Outport
  wires:
  theta/1 -> Mux5/2
  Mux6/1 -> x1y1/1
  Mux5/1 -> ->y2/1, ->x2/1
  x2y2/1 -> Mux5/1
  ->x2/1 -> Mux6/1
  ->y2/1 -> Mux6/2

== system SimplusGT/AC Infinite Bus (Current Type)/PQ Calculation (dq-Frame) ==
  note: Power calculation.
      |
      | Author(s): Yitong Li
      |
      | Notes:
      |
      | The calculation is done in dq frame.
  vdq : Inport
  idq : Inport  Port=2
  Mux : Mux  Inputs=2
  Mux1 : Mux  Inputs=2
  P = vd*id+vq*iq : Fcn  Expr=u[1]*u[3]+u[2]*u[4]
  Q = -vd*iq+vq*id : Fcn  Expr=-u[1]*u[4]+u[2]*u[3]
  pq : Outport
  wires:
  Q = -vd*iq+vq*id/1 -> Mux/2
  Mux1/1 -> Q = -vd*iq+vq*id/1, P = vd*id+vq*iq/1
  idq/1 -> Mux1/2
  vdq/1 -> Mux1/1
  P = vd*id+vq*iq/1 -> Mux/1
  Mux/1 -> pq/1

== system SimplusGT/AC Infinite Bus (Current Type)/abc -> dq (Power-Invariant) ==
  note: Frame transformation from abc to dq.
      |
      | Author(s): Yitong Li
      |
      | Notes:
      |
      | The transformation is power-invariant.
      |
      | theta is the angle that d axis leads a axis.
      |
      | q axis leads d axis by 90 degrees.
  abc : Inport
  theta : Inport  Port=2
  ->d : Fcn  Expr=cos(u(4))*u(1) + cos(u(4)-2/3*pi)*u(2) + cos(u(4)-4/3*pi)*u(3)
  ->q : Fcn  Expr=-sin(u(4))*u(1) - sin(u(4)-2/3*pi)*u(2) - sin(u(4)-4/3*pi)*u(3)
  Gain : Gain  Gain=sqrt(2/3)
  Mux5 : Mux  Inputs=2
  Mux6 : Mux  Inputs=2
  dq : Outport
  wires:
  Mux5/1 -> ->q/1, ->d/1
  Mux6/1 -> dq/1
  ->q/1 -> Mux6/2
  theta/1 -> Mux5/2
  Gain/1 -> Mux5/1
  ->d/1 -> Mux6/1
  abc/1 -> Gain/1

== system SimplusGT/AC Infinite Bus (Current Type)/dq -> abc (Power-Invariant) ==
  note: Frame transformation from dq to abc.
      |
      | Author(s): Yitong Li
      |
      | Notes:
      |
      | The transformation is power-invariant.
      |
      | theta is the angle that dq axis leads alpha/beta axis, specifically, d axis leads alpha axis.
  dq : Inport
  theta : Inport  Port=2
  ->a : Fcn  Expr=cos(u(3))*u(1) - sin(u(3))*u(2)
  ->b : Fcn  Expr=cos(u(3)-2/3*pi)*u(1) - sin(u(3)-2/3*pi)*u(2)
  ->c : Fcn  Expr=cos(u(3)-4/3*pi)*u(1) - sin(u(3)-4/3*pi)*u(2)
  Gain : Gain  Gain=sqrt(2/3)
  Mux5 : Mux  Inputs=2
  Mux6 : Mux  Inputs=3
  abc : Outport
  wires:
  theta/1 -> Mux5/2
  Mux5/1 -> ->c/1, ->a/1, ->b/1
  Mux6/1 -> abc/1
  ->c/1 -> Mux6/3
  dq/1 -> Gain/1
  Gain/1 -> Mux5/1
  ->a/1 -> Mux6/1
  ->b/1 -> Mux6/2

== system SimplusGT/AC Infinite Bus (Voltage Type)/PQ Calculation (dq-Frame)1 ==
  note: Power calculation.
      |
      | Author(s): Yitong Li
      |
      | Notes:
      |
      | The calculation is done in dq frame.
  vdq : Inport
  idq : Inport  Port=2
  Mux : Mux  Inputs=2
  Mux1 : Mux  Inputs=2
  P = vd*id+vq*iq : Fcn  Expr=u[1]*u[3]+u[2]*u[4]
  Q = -vd*iq+vq*id : Fcn  Expr=-u[1]*u[4]+u[2]*u[3]
  pq : Outport
  wires:
  Q = -vd*iq+vq*id/1 -> Mux/2
  Mux1/1 -> Q = -vd*iq+vq*id/1, P = vd*id+vq*iq/1
  idq/1 -> Mux1/2
  vdq/1 -> Mux1/1
  P = vd*id+vq*iq/1 -> Mux/1
  Mux/1 -> pq/1

== system SimplusGT/AC Infinite Bus (Voltage Type)/abc -> dq (Power-Invariant)1 ==
  note: Frame transformation from abc to dq.
      |
      | Author(s): Yitong Li
      |
      | Notes:
      |
      | The transformation is power-invariant.
      |
      | theta is the angle that d axis leads a axis.
      |
      | q axis leads d axis by 90 degrees.
  abc : Inport
  theta : Inport  Port=2
  ->d : Fcn  Expr=cos(u(4))*u(1) + cos(u(4)-2/3*pi)*u(2) + cos(u(4)-4/3*pi)*u(3)
  ->q : Fcn  Expr=-sin(u(4))*u(1) - sin(u(4)-2/3*pi)*u(2) - sin(u(4)-4/3*pi)*u(3)
  Gain : Gain  Gain=sqrt(2/3)
  Mux5 : Mux  Inputs=2
  Mux6 : Mux  Inputs=2
  dq : Outport
  wires:
  Mux5/1 -> ->q/1, ->d/1
  Mux6/1 -> dq/1
  ->q/1 -> Mux6/2
  theta/1 -> Mux5/2
  Gain/1 -> Mux5/1
  ->d/1 -> Mux6/1
  abc/1 -> Gain/1

== system SimplusGT/AC Infinite Bus (Voltage Type)/dq -> abc (Power-Invariant)1 ==
  note: Frame transformation from dq to abc.
      |
      | Author(s): Yitong Li
      |
      | Notes:
      |
      | The transformation is power-invariant.
      |
      | theta is the angle that dq axis leads alpha/beta axis, specifically, d axis leads alpha axis.
  dq : Inport
  theta : Inport  Port=2
  ->a : Fcn  Expr=cos(u(3))*u(1) - sin(u(3))*u(2)
  ->b : Fcn  Expr=cos(u(3)-2/3*pi)*u(1) - sin(u(3)-2/3*pi)*u(2)
  ->c : Fcn  Expr=cos(u(3)-4/3*pi)*u(1) - sin(u(3)-4/3*pi)*u(2)
  Gain : Gain  Gain=sqrt(2/3)
  Mux5 : Mux  Inputs=2
  Mux6 : Mux  Inputs=3
  abc : Outport
  wires:
  theta/1 -> Mux5/2
  Mux5/1 -> ->c/1, ->a/1, ->b/1
  Mux6/1 -> abc/1
  ->c/1 -> Mux6/3
  dq/1 -> Gain/1
  Gain/1 -> Mux5/1
  ->a/1 -> Mux6/1
  ->b/1 -> Mux6/2

== system SimplusGT/Battery (dq-Frame System Object)/PQ Calculation (dq-Frame) ==
  note: Power calculation.
      |
      | Author(s): Yitong Li
      |
      | Notes:
      |
      | The calculation is done in dq frame.
  vdq : Inport
  idq : Inport  Port=2
  Mux : Mux  Inputs=2
  Mux1 : Mux  Inputs=2
  P = vd*id+vq*iq : Fcn  Expr=u[1]*u[3]+u[2]*u[4]
  Q = -vd*iq+vq*id : Fcn  Expr=-u[1]*u[4]+u[2]*u[3]
  pq : Outport
  wires:
  Mux/1 -> pq/1
  P = vd*id+vq*iq/1 -> Mux/1
  vdq/1 -> Mux1/1
  idq/1 -> Mux1/2
  Mux1/1 -> P = vd*id+vq*iq/1, Q = -vd*iq+vq*id/1
  Q = -vd*iq+vq*id/1 -> Mux/2

== system SimplusGT/Battery (dq-Frame System Object)/abc -> dq (Power-Invariant) ==
  note: Frame transformation from abc to dq.
      |
      | Author(s): Yitong Li
      |
      | Notes:
      |
      | The transformation is power-invariant.
      |
      | theta is the angle that d axis leads a axis.
      |
      | q axis leads d axis by 90 degrees.
  abc : Inport
  theta : Inport  Port=2
  ->d : Fcn  Expr=cos(u(4))*u(1) + cos(u(4)-2/3*pi)*u(2) + cos(u(4)-4/3*pi)*u(3)
  ->q : Fcn  Expr=-sin(u(4))*u(1) - sin(u(4)-2/3*pi)*u(2) - sin(u(4)-4/3*pi)*u(3)
  Gain : Gain  Gain=sqrt(2/3)
  Mux5 : Mux  Inputs=2
  Mux6 : Mux  Inputs=2
  dq : Outport
  wires:
  abc/1 -> Gain/1
  ->d/1 -> Mux6/1
  Gain/1 -> Mux5/1
  theta/1 -> Mux5/2
  ->q/1 -> Mux6/2
  Mux6/1 -> dq/1
  Mux5/1 -> ->d/1, ->q/1

== system SimplusGT/Battery (dq-Frame System Object)/abc -> dq (Power-Invariant)1 ==
  note: Frame transformation from abc to dq.
      |
      | Author(s): Yitong Li
      |
      | Notes:
      |
      | The transformation is power-invariant.
      |
      | theta is the angle that d axis leads a axis.
      |
      | q axis leads d axis by 90 degrees.
  abc : Inport
  theta : Inport  Port=2
  ->d : Fcn  Expr=cos(u(4))*u(1) + cos(u(4)-2/3*pi)*u(2) + cos(u(4)-4/3*pi)*u(3)
  ->q : Fcn  Expr=-sin(u(4))*u(1) - sin(u(4)-2/3*pi)*u(2) - sin(u(4)-4/3*pi)*u(3)
  Gain : Gain  Gain=sqrt(2/3)
  Mux5 : Mux  Inputs=2
  Mux6 : Mux  Inputs=2
  dq : Outport
  wires:
  abc/1 -> Gain/1
  ->d/1 -> Mux6/1
  Gain/1 -> Mux5/1
  theta/1 -> Mux5/2
  ->q/1 -> Mux6/2
  Mux6/1 -> dq/1
  Mux5/1 -> ->d/1, ->q/1

== system SimplusGT/Battery (dq-Frame System Object)/dq -> abc (Power-Invariant) ==
  note: Frame transformation from dq to abc.
      |
      | Author(s): Yitong Li
      |
      | Notes:
      |
      | The transformation is power-invariant.
      |
      | theta is the angle that dq axis leads alpha/beta axis, specifically, d axis leads alpha axis.
  dq : Inport
  theta : Inport  Port=2
  ->a : Fcn  Expr=cos(u(3))*u(1) - sin(u(3))*u(2)
  ->b : Fcn  Expr=cos(u(3)-2/3*pi)*u(1) - sin(u(3)-2/3*pi)*u(2)
  ->c : Fcn  Expr=cos(u(3)-4/3*pi)*u(1) - sin(u(3)-4/3*pi)*u(2)
  Gain : Gain  Gain=sqrt(2/3)
  Mux5 : Mux  Inputs=2
  Mux6 : Mux  Inputs=3
  abc : Outport
  wires:
  ->b/1 -> Mux6/2
  ->a/1 -> Mux6/1
  Gain/1 -> Mux5/1
  dq/1 -> Gain/1
  ->c/1 -> Mux6/3
  Mux6/1 -> abc/1
  Mux5/1 -> ->b/1, ->a/1, ->c/1
  theta/1 -> Mux5/2

== system SimplusGT/Frequency Droop (iDQ -> id)/x1y1 -> x2y2 ==
  note: Frame transformation from x1y1 to x2y2.
      |
      | Author(s): Yitong Li
      |
      | Notes:
      |
      | theta is the phase angle that coordinate 2 (axis) leads coordinate 1 (axis).
  x1y1 : Inport
  theta : Inport  Port=2
  ->x2 : Fcn  Expr=cos(u(3))*u(1) + sin(u(3))*u(2)
  ->y2 : Fcn  Expr=-sin(u(3))*u(1) + cos(u(3))*u(2)
  Mux5 : Mux  Inputs=2
  Mux6 : Mux  Inputs=2
  x2y2 : Outport
  wires:
  ->x2/1 -> Mux6/1
  ->y2/1 -> Mux6/2
  x1y1/1 -> Mux5/1
  theta/1 -> Mux5/2
  Mux5/1 -> ->x2/1, ->y2/1
  Mux6/1 -> x2y2/1

== system SimplusGT/Frequency Droop (iabc -> id)/abc -> dq (Power-Invariant) ==
  note: Frame transformation from abc to dq.
      |
      | Author(s): Yitong Li
      |
      | Notes:
      |
      | The transformation is power-invariant.
      |
      | theta is the angle that d axis leads a axis.
      |
      | q axis leads d axis by 90 degrees.
  abc : Inport
  theta : Inport  Port=2
  ->d : Fcn  Expr=cos(u(4))*u(1) + cos(u(4)-2/3*pi)*u(2) + cos(u(4)-4/3*pi)*u(3)
  ->q : Fcn  Expr=-sin(u(4))*u(1) - sin(u(4)-2/3*pi)*u(2) - sin(u(4)-4/3*pi)*u(3)
  Gain : Gain  Gain=sqrt(2/3)
  Mux5 : Mux  Inputs=2
  Mux6 : Mux  Inputs=2
  dq : Outport
  wires:
  abc/1 -> Gain/1
  ->d/1 -> Mux6/1
  Gain/1 -> Mux5/1
  theta/1 -> Mux5/2
  ->q/1 -> Mux6/2
  Mux6/1 -> dq/1
  Mux5/1 -> ->d/1, ->q/1

== system SimplusGT/Frequency Droop (iabc -> id+jiq)/abc -> dq (Power-Invariant)1 ==
  note: Frame transformation from abc to dq.
      |
      | Author(s): Yitong Li
      |
      | Notes:
      |
      | The transformation is power-invariant.
      |
      | theta is the angle that d axis leads a axis.
      |
      | q axis leads d axis by 90 degrees.
  abc : Inport
  theta : Inport  Port=2
  ->d : Fcn  Expr=cos(u(4))*u(1) + cos(u(4)-2/3*pi)*u(2) + cos(u(4)-4/3*pi)*u(3)
  ->q : Fcn  Expr=-sin(u(4))*u(1) - sin(u(4)-2/3*pi)*u(2) - sin(u(4)-4/3*pi)*u(3)
  Gain : Gain  Gain=sqrt(2/3)
  Mux5 : Mux  Inputs=2
  Mux6 : Mux  Inputs=2
  dq : Outport
  wires:
  abc/1 -> Gain/1
  ->d/1 -> Mux6/1
  Gain/1 -> Mux5/1
  theta/1 -> Mux5/2
  ->q/1 -> Mux6/2
  Mux6/1 -> dq/1
  Mux5/1 -> ->d/1, ->q/1

== system SimplusGT/Frequency Droop (iabc -> iq)/abc -> dq (Power-Invariant)1 ==
  note: Frame transformation from abc to dq.
      |
      | Author(s): Yitong Li
      |
      | Notes:
      |
      | The transformation is power-invariant.
      |
      | theta is the angle that d axis leads a axis.
      |
      | q axis leads d axis by 90 degrees.
  abc : Inport
  theta : Inport  Port=2
  ->d : Fcn  Expr=cos(u(4))*u(1) + cos(u(4)-2/3*pi)*u(2) + cos(u(4)-4/3*pi)*u(3)
  ->q : Fcn  Expr=-sin(u(4))*u(1) - sin(u(4)-2/3*pi)*u(2) - sin(u(4)-4/3*pi)*u(3)
  Gain : Gain  Gain=sqrt(2/3)
  Mux5 : Mux  Inputs=2
  Mux6 : Mux  Inputs=2
  dq : Outport
  wires:
  abc/1 -> Gain/1
  ->d/1 -> Mux6/1
  Gain/1 -> Mux5/1
  theta/1 -> Mux5/2
  ->q/1 -> Mux6/2
  Mux6/1 -> dq/1
  Mux5/1 -> ->d/1, ->q/1

== system SimplusGT/Grid-Following Voltage-Source Inverter (dq-Frame System Object)/PQ Calculation (dq-Frame)1 ==
  note: Power calculation.
      |
      | Author(s): Yitong Li
      |
      | Notes:
      |
      | The calculation is done in dq frame.
  vdq : Inport
  idq : Inport  Port=2
  Mux : Mux  Inputs=2
  Mux1 : Mux  Inputs=2
  P = vd*id+vq*iq : Fcn  Expr=u[1]*u[3]+u[2]*u[4]
  Q = -vd*iq+vq*id : Fcn  Expr=-u[1]*u[4]+u[2]*u[3]
  pq : Outport
  wires:
  Q = -vd*iq+vq*id/1 -> Mux/2
  Mux1/1 -> Q = -vd*iq+vq*id/1, P = vd*id+vq*iq/1
  idq/1 -> Mux1/2
  vdq/1 -> Mux1/1
  P = vd*id+vq*iq/1 -> Mux/1
  Mux/1 -> pq/1

== system SimplusGT/Grid-Following Voltage-Source Inverter (dq-Frame System Object)/abc -> dq (Power-Invariant)1 ==
  note: Frame transformation from abc to dq.
      |
      | Author(s): Yitong Li
      |
      | Notes:
      |
      | The transformation is power-invariant.
      |
      | theta is the angle that d axis leads a axis.
      |
      | q axis leads d axis by 90 degrees.
  abc : Inport
  theta : Inport  Port=2
  ->d : Fcn  Expr=cos(u(4))*u(1) + cos(u(4)-2/3*pi)*u(2) + cos(u(4)-4/3*pi)*u(3)
  ->q : Fcn  Expr=-sin(u(4))*u(1) - sin(u(4)-2/3*pi)*u(2) - sin(u(4)-4/3*pi)*u(3)
  Gain : Gain  Gain=sqrt(2/3)
  Mux5 : Mux  Inputs=2
  Mux6 : Mux  Inputs=2
  dq : Outport
  wires:
  Mux5/1 -> ->q/1, ->d/1
  Mux6/1 -> dq/1
  ->q/1 -> Mux6/2
  theta/1 -> Mux5/2
  Gain/1 -> Mux5/1
  ->d/1 -> Mux6/1
  abc/1 -> Gain/1

== system SimplusGT/Grid-Following Voltage-Source Inverter (dq-Frame System Object)/abc -> dq (Power-Invariant)2 ==
  note: Frame transformation from abc to dq.
      |
      | Author(s): Yitong Li
      |
      | Notes:
      |
      | The transformation is power-invariant.
      |
      | theta is the angle that d axis leads a axis.
      |
      | q axis leads d axis by 90 degrees.
  abc : Inport
  theta : Inport  Port=2
  ->d : Fcn  Expr=cos(u(4))*u(1) + cos(u(4)-2/3*pi)*u(2) + cos(u(4)-4/3*pi)*u(3)
  ->q : Fcn  Expr=-sin(u(4))*u(1) - sin(u(4)-2/3*pi)*u(2) - sin(u(4)-4/3*pi)*u(3)
  Gain : Gain  Gain=sqrt(2/3)
  Mux5 : Mux  Inputs=2
  Mux6 : Mux  Inputs=2
  dq : Outport
  wires:
  Mux5/1 -> ->q/1, ->d/1
  Mux6/1 -> dq/1
  ->q/1 -> Mux6/2
  theta/1 -> Mux5/2
  Gain/1 -> Mux5/1
  ->d/1 -> Mux6/1
  abc/1 -> Gain/1

== system SimplusGT/Grid-Following Voltage-Source Inverter (dq-Frame System Object)/dq -> abc (Power-Invariant)1 ==
  note: Frame transformation from dq to abc.
      |
      | Author(s): Yitong Li
      |
      | Notes:
      |
      | The transformation is power-invariant.
      |
      | theta is the angle that dq axis leads alpha/beta axis, specifically, d axis leads alpha axis.
  dq : Inport
  theta : Inport  Port=2
  ->a : Fcn  Expr=cos(u(3))*u(1) - sin(u(3))*u(2)
  ->b : Fcn  Expr=cos(u(3)-2/3*pi)*u(1) - sin(u(3)-2/3*pi)*u(2)
  ->c : Fcn  Expr=cos(u(3)-4/3*pi)*u(1) - sin(u(3)-4/3*pi)*u(2)
  Gain : Gain  Gain=sqrt(2/3)
  Mux5 : Mux  Inputs=2
  Mux6 : Mux  Inputs=3
  abc : Outport
  wires:
  theta/1 -> Mux5/2
  Mux5/1 -> ->c/1, ->a/1, ->b/1
  Mux6/1 -> abc/1
  ->c/1 -> Mux6/3
  dq/1 -> Gain/1
  Gain/1 -> Mux5/1
  ->a/1 -> Mux6/1
  ->b/1 -> Mux6/2

== system SimplusGT/Grid-Following Inverter (Simulink Block)/Current Controller ==
  iIdq* : Inport
  iIdq : Inport  Port=2
  vdq : Inport  Port=3
  enable : Inport  Port=4
  Constant : Constant  Value=Kcd
  Demux1 : Demux  Outputs=2
  Demux2 : Demux  Outputs=2
  Demux3 : Demux  Outputs=2
  Mux : Mux  Inputs=2
  PI-DT-Estimated d : Subsystem  mask{Lf=Lf, Kg=Kg, Kp=Kp, Ki=Ki, xmax=vdmax, xmin=-vdmax, Ts=Ts}
      mask prompts: Lf "Inductance"; Kg "Estimator Gain"; Kp "Proportional Gain"; Ki "Integral Gain"; xmax "Upper Limit"; xmin "Lower Limit"; Ts "Sampling Time"
  PI-DT-Estimated q : Subsystem  mask{Lf=Lf, Kg=Kg, Kp=Kp, Ki=Ki, xmax=vqmax, xmin=-vqmax, Ts=Ts}
      mask prompts: Lf "Inductance"; Kg "Estimator Gain"; Kp "Proportional Gain"; Ki "Integral Gain"; xmax "Upper Limit"; xmin "Lower Limit"; Ts "Sampling Time"
  Product : Product
  Product1 : Product
  sum_d : Sum  Inputs=+-
  sum_q : Sum
  wLd : Gain  Gain=Wbase*Lf
  wLq : Gain  Gain=Wbase*Lf
  vidq* : Outport
  wires:
  sum_d/1 -> Mux/1
  sum_q/1 -> Mux/2
  iIdq/1 -> Demux1/1
  Demux1/1 -> wLd/1, PI-DT-Estimated d/4(actual)
  Demux1/2 -> PI-DT-Estimated q/1(actual), wLq/1
  Mux/1 -> vidq*/1
  PI-DT-Estimated d/1(Out) -> sum_d/1
  vdq/1 -> Demux3/1
  PI-DT-Estimated q/1(Out) -> sum_q/2
  Demux3/2 -> PI-DT-Estimated q/2(initial)
  Demux3/1 -> PI-DT-Estimated d/3(initial)
  iIdq*/1 -> Demux2/1
  Demux2/1 -> PI-DT-Estimated d/2(reference)
  Demux2/2 -> PI-DT-Estimated q/3(reference)
  enable/1 -> PI-DT-Estimated q/4(enable), PI-DT-Estimated d/1(enable)
  wLd/1 -> Product/1
  Product/1 -> sum_q/1
  wLq/1 -> Product1/2
  Product1/1 -> sum_d/2
  Constant/1 -> Product/2, Product1/1
